simulink model "DynamicSubsystem"  (R2022b)
settings: Solver=ode45  StartTime=0.0  StopTime=20  RelTol=1e-3
settings Model: Creator=Mo_7atem  LastModifiedBy=Mo_7atem

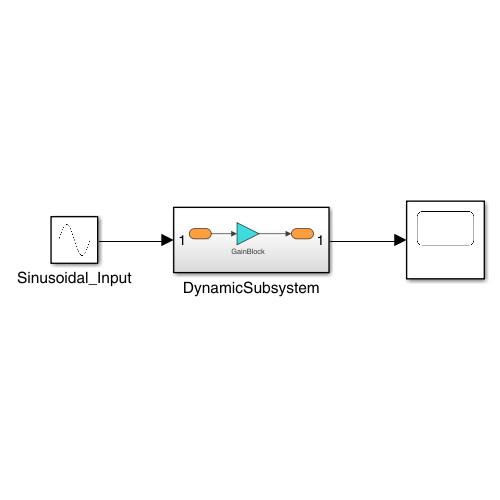
[thumbnail: Simulink's stored preview of the top-level diagram]
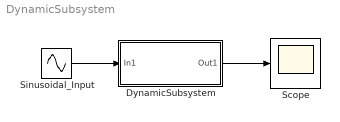
== system DynamicSubsystem ==
  DynamicSubsystem : Subsystem
  Scope : Scope
  Sinusoidal_Input : Sin  SampleTime=0
  wires:
  Sinusoidal_Input/1 -> DynamicSubsystem/1(In1)
  DynamicSubsystem/1(Out1) -> Scope/1

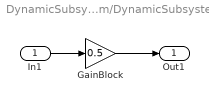
== system DynamicSubsystem/DynamicSubsystem ==
  In1 : Inport
  GainBlock : Gain  Gain=0.5
  Out1 : Outport
  wires:
  In1/1 -> GainBlock/1
  GainBlock/1 -> Out1/1
